simulink model "SVM_test2"  (R2020a)
settings: Solver=VariableStepAuto  StartTime=0.0  StopTime=Inf  FixedStep=Ts/2  RelTol=1e-3
PostLoadFcn:
  | , if any(exist('dsrtsu_mdlpostloadfcn', 'file') ~= 0), dsrtsu_mdlpostloadfcn('Execute', bdroot); end,
InitFcn:
  | , if any(exist('rtifpga_mdlclblib', 'file') ~= 0), rtifpga_mdlclblib('Init', bdroot); end,
model workspace (MAT data in the model file):
  FPGA_SVM_test2_1_Register_1_1_1_write = Simulink.Signal
  FPGA_SVM_test2_1_Register_1_1_1_write.Description = 'RTIFPGA'
  FPGA_SVM_test2_1_Register_1_1_1_write.DataType = 'double'
  FPGA_SVM_test2_1_Register_1_1_1_write.Dimensions = '1'
  FPGA_SVM_test2_1_Register_1_1_1_write.DimensionsMode = 'auto'
  FPGA_SVM_test2_1_Register_1_1_1_write.Complexity = 'auto'
  FPGA_SVM_test2_1_Register_1_1_1_write.SampleTime = -1
  FPGA_SVM_test2_1_Register_1_1_1_write.SamplingMode = 'auto'
  FPGA_SVM_test2_1_Register_2_1_1_write = Simulink.Signal
  FPGA_SVM_test2_1_Register_2_1_1_write.Description = 'RTIFPGA'
  FPGA_SVM_test2_1_Register_2_1_1_write.DataType = 'double'
  FPGA_SVM_test2_1_Register_2_1_1_write.Dimensions = '1'
  FPGA_SVM_test2_1_Register_2_1_1_write.DimensionsMode = 'auto'
  FPGA_SVM_test2_1_Register_2_1_1_write.Complexity = 'auto'
  FPGA_SVM_test2_1_Register_2_1_1_write.SampleTime = -1
  FPGA_SVM_test2_1_Register_2_1_1_write.SamplingMode = 'auto'
  FPGA_SVM_test2_1_Register_3_1_1_write = Simulink.Signal
  FPGA_SVM_test2_1_Register_3_1_1_write.Description = 'RTIFPGA'
  FPGA_SVM_test2_1_Register_3_1_1_write.DataType = 'double'
  FPGA_SVM_test2_1_Register_3_1_1_write.Dimensions = '1'
  FPGA_SVM_test2_1_Register_3_1_1_write.DimensionsMode = 'auto'
  FPGA_SVM_test2_1_Register_3_1_1_write.Complexity = 'auto'
  FPGA_SVM_test2_1_Register_3_1_1_write.SampleTime = -1
  FPGA_SVM_test2_1_Register_3_1_1_write.SamplingMode = 'auto'
  FPGA_SVM_test2_1_Register_4_1_1_write = Simulink.Signal
  FPGA_SVM_test2_1_Register_4_1_1_write.Description = 'RTIFPGA'
  FPGA_SVM_test2_1_Register_4_1_1_write.DataType = 'double'
  FPGA_SVM_test2_1_Register_4_1_1_write.Dimensions = '1'
  FPGA_SVM_test2_1_Register_4_1_1_write.DimensionsMode = 'auto'
  FPGA_SVM_test2_1_Register_4_1_1_write.Complexity = 'auto'
  FPGA_SVM_test2_1_Register_4_1_1_write.SampleTime = -1
  FPGA_SVM_test2_1_Register_4_1_1_write.SamplingMode = 'auto'
  FPGA_SVM_test2_1_Register_5_1_1_write = Simulink.Signal
  FPGA_SVM_test2_1_Register_5_1_1_write.Description = 'RTIFPGA'
  FPGA_SVM_test2_1_Register_5_1_1_write.DataType = 'double'
  FPGA_SVM_test2_1_Register_5_1_1_write.Dimensions = '1'
  FPGA_SVM_test2_1_Register_5_1_1_write.DimensionsMode = 'auto'
  FPGA_SVM_test2_1_Register_5_1_1_write.Complexity = 'auto'
  FPGA_SVM_test2_1_Register_5_1_1_write.SampleTime = -1
  FPGA_SVM_test2_1_Register_5_1_1_write.SamplingMode = 'auto'
  FPGA_SVM_test2_1_Register_6_1_1_write = Simulink.Signal
  FPGA_SVM_test2_1_Register_6_1_1_write.Description = 'RTIFPGA'
  FPGA_SVM_test2_1_Register_6_1_1_write.DataType = 'double'
  FPGA_SVM_test2_1_Register_6_1_1_write.Dimensions = '1'
  FPGA_SVM_test2_1_Register_6_1_1_write.DimensionsMode = 'auto'
  FPGA_SVM_test2_1_Register_6_1_1_write.Complexity = 'auto'
  FPGA_SVM_test2_1_Register_6_1_1_write.SampleTime = -1
  FPGA_SVM_test2_1_Register_6_1_1_write.SamplingMode = 'auto'
  FPGA_SVM_test2_1_Register_7_1_1_write = Simulink.Signal
  FPGA_SVM_test2_1_Register_7_1_1_write.Description = 'RTIFPGA'
  FPGA_SVM_test2_1_Register_7_1_1_write.DataType = 'double'
  FPGA_SVM_test2_1_Register_7_1_1_write.Dimensions = '1'
  FPGA_SVM_test2_1_Register_7_1_1_write.DimensionsMode = 'auto'
  FPGA_SVM_test2_1_Register_7_1_1_write.Complexity = 'auto'
  FPGA_SVM_test2_1_Register_7_1_1_write.SampleTime = -1
  FPGA_SVM_test2_1_Register_7_1_1_write.SamplingMode = 'auto'
values from neighbouring files (symbols this model uses):
  clamp_threshold = 400    [param.m]
  i_fixed_gain = 10*1000/(3*100)    (= 33.3333333333)    [param.m]
  ioa_gain = 1    [param.m]
  ioa_offset = 0.09    [param.m]
  iob_gain = 1    [param.m]
  iob_offset = 0.06    [param.m]
  isa_gain = 1    [param.m]
  isa_offset = 0.1    [param.m]
  isb_gain = 1    [param.m]
  isb_offset = 0.3    [param.m]
  N = 1000    [param.m]
  vca_gain = 1    [param.m]
  vca_offset = 0.8    [param.m]
  vcb_gain = 1    [param.m]
  vcb_offset = 1.7    [param.m]
  vcc_gain = 1    [param.m]
  vcc_offset = 3    [param.m]
  vclamp_gain = 10*(76000+47000)/(3*100*2.5)    (= 1640)    [param.m]
  vclamp_offset = 11.7    [param.m]
  vi_fixed_gain = 10*33000/(3*100*2.5)    (= 440)    [param.m]
  via_gain = 1    [param.m]
  via_offset = 1    [param.m]
  vib_gain = 1    [param.m]
  vib_offset = 0.8    [param.m]
  vic_gain = 1    [param.m]
  vic_offset = -0.35    [param.m]
  voa_fixed_gain = 10*30000/(3*100*2.5)    (= 400)    [param.m]
  voa_gain = 1    [param.m]
  voa_offset = 0.7    [param.m]
libraries: xbsIndex_r4 x466, rti1202lib_adc_class1 x12, rtiproclib x10, simulink x3, rtifpgainterfacelib x1, powerlib_meascontrol x1
(part 1 of 9)
Description:
  | Standard RTI1202 template.
  | Supported MATLAB version:  R2020a.
settings Model: Tag=RTI1202  DSRTSU_INTERNAL_RTI_VER=570  DSRTSU_INTERNAL_RTI_TYPE=rti1202  RTICANMMDATA=struct('GeneralSetupData',struct('modelroot','D:\MarcosGomez\SVM','generalsettings',struct('filesettings',struct('destfolder',struct('Name','RTICANMM_FILES','Check',1),'buildfolder',struct('Name','.','Check',1),'AbsDestfolder',struct('Name','D:\MarcosGomez\SVM\RTICANMM_FILES'),'AbsBuildfolder',struct('Name','D:\MarcosGomez\SVM'))),'options',struct('addpaths',1,'rmpaths',1,'addtrcexclusion',true,'cannavigator',struct('checkmonitoring',0),'show_usrtrc',0,'use_usrtrc',0),'advanced',struct('options',ones(1,100)),'MPSetup',{{}},'RTI',struct('Type','RTI1202','Ver','7.15','Date','02-Nov-2020'),'modelname','SVM_test2','block','SVM_test2'))  DSRTSU_INTERNAL_RTIFPGA=170  OrderedModelArguments=off  Creator=dSPACE2023A  LastModifiedBy=dspace
settings DataIOCC: ReturnWorkspaceOutputs=off
settings OptimizationCC: BlockReduction=off  OptimizeBlockIOStorage=off  BufferReuse=off  GlobalBufferReuse=off  ExpressionFolding=off  LocalBlockOutputs=off  OptimizeDataStoreBuffers=off  BusAssignmentInplaceUpdate=off
settings DebuggingCC: PregeneratedLibrarySubsystemCodeDiagnostic=none  ArithmeticOperatorsInVariantConditions=warning
settings HardwareCC: ProdBitPerPointer=32  ProdBitPerSizeT=32  ProdBitPerPtrDiffT=32  ProdLargestAtomicInteger=Integer  ProdEndianess=BigEndian  ProdWordSize=32  ProdLongLongMode=on  ProdHWDeviceType=Custom Processor->Custom  TargetIntDivRoundTo=Zero  TargetEndianess=BigEndian  TargetHWDeviceType=Custom Processor->Custom
settings ModelReferenceCC: EnableParallelModelReferenceBuilds=on  ParallelModelReferenceMATLABWorkerInit=Load Top Model
settings SFSimCC: SimUseLocalCustomCode=off  MATLABDynamicMemAlloc=off  CustomCodeUndefinedFunction=UseInterfaceOnly
settings RTWCC: Description=dSPACE DS1202 Hardware Platform  SystemTargetFile=rti1202.tlc  MakeCommand=make_rti  TemplateMakefile=rti1202.tmf  RTWUseLocalCustomCode=off
settings CodeAppCC: StateflowObjectComments=on
settings STFCustomTargetCC: ParMdlRefBuildCompliant=on  SystemTargetFile=rti1202.tlc
settings GRTTargetCC: TargetLangStandard=C89/C90 (ANSI)  CompOptLevelCompliant=off  ConcurrentExecutionCompliant=off  CombineOutputUpdateFcns=off  MatFileLogging=off  CPPClassGenCompliant=off  UseToolchainInfoCompliant=off
settings ConfigComp: CovMetricSettings=dswe

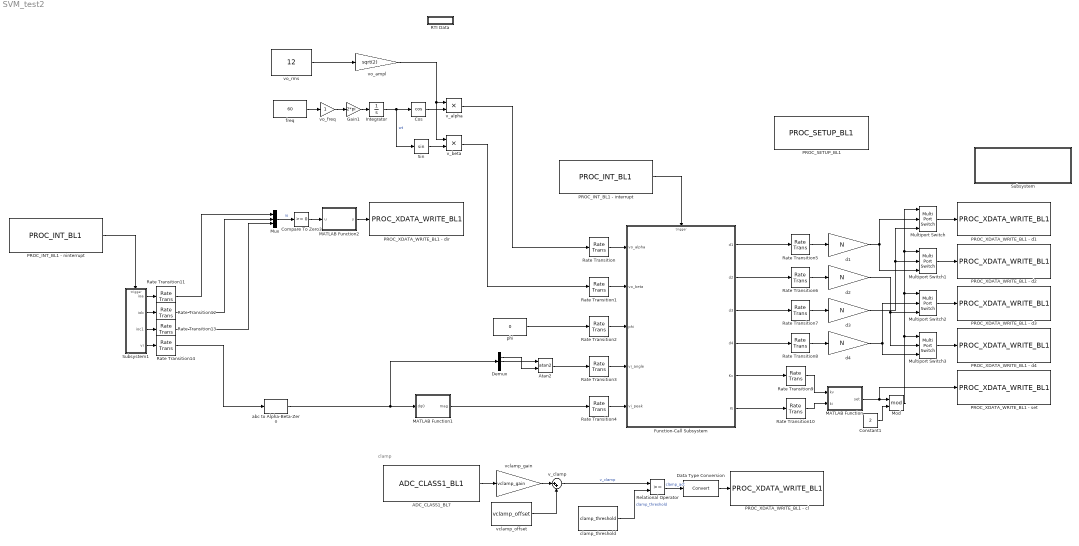
== system SVM_test2 ==
  note: clamp
  ADC_CLASS1_BL7 : rti1202lib_adc_class1/ADC_CLASS1_BL1  DSProperties=struct('RTI',struct('Version',uint32(1),'BlockType',struct('isSLSource',uint8(1),'isSLSink',uint8(1),'isHWSource',uint8(0),'isHWSink',uint8(1),'isSetup',uint8(0),'isInline',uint8(1),'isNonInline',uint8(0),'isInterrupt',uint8(0),'isChannelwise',uint8(1)),'IOBoardType',{{'DS120X','STD','ADCC1'}},'UnitType','ADC','Identifier','ADC','DialogType','ML','BlockSet','NONE','SlaveProcessor','NONE'))  RTIBlockInterface=struct('InputPortsActive',0,'InputPortsWidth',int32(1),'InputPortsDataType',{{'SS_BOOLEAN'}},'InputPortsName',{{'Continue'}},'OutputPortsActive',[1 0],'OutputPortsWidth',int32([1 1]),'OutputPortsDataType',{{'SS_DOUBLE','SS_INT16'}},'OutputPortsName',{{'ADC','Status'}},'DialogFcn','rti120xstdadcc1adcgui','SampleTime',{{-1}},'InitLevel',3,'IconTransparency','on','BlockDisplay',{{['ADC CL1\nChannel: 7'],'center'}},'BlockName',struct('Token',{{'ADC_CLASS1_BL1'}}))  RTIBlockParameters=struct('ReadMode',{{1,'OFF',[1 2]}},'ChannelNo',{{7,'OFF',[]}},'ConversionMode',{{1,'OFF',[1 2]}},'TriggerSource',{{1,'OFF',[1 2]}},'TriggerLineIn',{{1,'OFF',[1 16]}},'SampleMode',{{1,'OFF',[1 2]}},'BurstTriggerSource',{{1,'OFF',[1 2]}},'BurstTriggerLine',{{1,'OFF',[1 16]}},'ConvTriggerSource',{{3,'OFF',[1 3]}},'ConvTriggerLine',{{1,'OFF',[1 16]}},'ConvPeriod',{{'100e-6','OFF',[1e-6 1.34]}},'ConvPeriodCheck',{{0,'OFF',[]}},'BurstSize',{{'10','OFF',[]}},'BurstSizeCheck',{{0,'OFF',[]}},'DataSetOffset',{{'0','OFF',[]}},'DataSetOffsetCheck',{{0,'OFF',[]}},'DataSetLength',{{'1','OFF',[]}},'DataSetLengthCheck',{{0,'OFF',[]}},'EnableTriggerEvent',{{0,'OFF',[0 1]}},'TriggerMode',{{2,'OFF',[1 3]}},'TriggerLineOut',{{1,'OFF',[1 16]}},'ADCSWStartEnable',{{0,'OFF',[0 1]}},'SampleTime',{{'-1','OFF',[-1 inf]}},'SampleTimeCheck',{{1,'OFF',[]}},'StatusPortEnable',{{0,'OFF',[0 1]}},'TLCFileName',{{'rti120xadc_c1_adc','OFF',[]}})  RTISFcnParameters=struct('ReadMode','int16','ChannelNo','int16','ConversionMode','int16','TriggerSource','int16','TriggerLineIn','int16','SampleMode','int16','BurstTriggerSource','int16','BurstTriggerLine','int16','ConvTriggerSource','int16','ConvTriggerLine','int16','ConvPeriod','double','BurstSize','int16','DataSetOffset','int16','DataSetLength','int16','EnableTriggerEvent','int16','TriggerMode','int16','TriggerLineOut','int16','ADCSWStartEnable','int16','SampleTime','double','StatusPortEnable','int16','TLCFileName','char')  RTIBlockParaDefault=struct('ReadMode',1,'ChannelNo',1,'ConversionMode',1,'TriggerSource',1,'TriggerLineIn',1,'SampleMode',1,'BurstTriggerSource',1,'BurstTriggerLine',1,'ConvTriggerSource',3,'ConvTriggerLine',1,'ConvPeriod',0.0001,'ConvPeriodCheck',0,'BurstSize',10,'BurstSizeCheck',0,'DataSetOffset',0,'DataSetOffsetCheck',0,'DataSetLength',1,'DataSetLengthCheck',0,'EnableTriggerEvent',0,'TriggerMode',2,'TriggerLineOut',1,'ADCSWStartEnable',0,'SampleTime',-1,'SampleTimeCheck',1,'StatusPortEnable',0,'TLCFileName','rti120xadc_c1_adc')
  Atan2 : Trigonometry  Operator=atan2
  Compare To Zero3 : simulink/Logic and Bit Operations/Compare To Zero  relop=>=  OutDataTypeStr=boolean
  Constant1 : Constant  Value=2
  Cos : Trigonometry  Operator=cos
  Data Type Conversion : DataTypeConversion
  Demux : Demux  Outputs=3
  Function-Call Subsystem : Subsystem  TreatAsAtomicUnit=on
  Gain1 : Gain  Gain=2*pi
  Integrator : Integrator
  MATLAB Function : MATLAB Function  TreatAsAtomicUnit=on
  MATLAB Function1 : MATLAB Function  TreatAsAtomicUnit=on
  MATLAB Function2 : MATLAB Function  TreatAsAtomicUnit=on
  Mod : Math  Operator=mod  SaturateOnIntegerOverflow=on
  Multiport Switch{,1..3} (4 alike) : MultiPortSwitch  DataPortOrder=Zero-based contiguous  Inputs=2  zeroidx=on
  Mux : Mux  Inputs=3
  PROC_INT_BL1 - interrupt : rtiproclib/PROC_INT_BL1  DSProperties=struct('RTI',struct('Version',uint32(4),'BlockType',struct('isSLSource',uint8(1),'isSLSink',uint8(0),'isHWSource',uint8(0),'isHWSink',uint8(0),'isSetup',uint8(1),'isInline',uint8(1),'isNonInline',uint8(0),'isInterrupt',uint8(0),'isChannelwise',uint8(0)),'IOBoardType','DSPROC','UnitType','','Identifier','INT','DialogType','ML','BlockSet','DSPROC','SlaveProcessor',''))  RTIBlockInterface=struct('OutputPortsActive',1,'OutputPortsWidth',int32(1),'OutputPortsName',{{'Interrupt'}},'FunctionCall',uint32(0),'DialogFcn','rtiprocintgui','InitLevel',3,'BlockDisplay',{{['Interrupt In 1\ninterrupt \nBoard: 1'],'center'}},'IconTransparency','on','BlockName',struct('Token',{{'PROC_INT_BL1'}}))  RTIBlockParameters=struct('BoardNo',{{'1','OFF',[1 16]}},'ChannelNo',{{'1','OFF',[1 8]}},'AccessTyp',{{'Interrupt','OFF',[]}},'BinaryPoint',{{'0','OFF',[]}},'DataFormat',{{'unsigned','OFF',[]}},'BufferLength',{{'0','OFF',[]}},'MultiChAccess',{{'0','OFF',[]}},'ModelPortBlock',{{{struct('BlockId','','SignalId','')},'OFF',[]}})  RTISFcnParameters=struct('BoardNo','double','ChannelNo','double','AccessTyp','char','BinaryPoint','double','DataFormat','char','BufferLength','double')  RTIBlockParaDefault=struct('BoardNo','1','ChannelNo','1','AccessTyp','Interrupt','BinaryPoint','10','DataFormat','unsigned','BufferLength','0','MultiChAccess','0','ModelPortBlock',{{struct('BlockId','','SignalId','')}})
  PROC_INT_BL1 - ninterrupt : rtiproclib/PROC_INT_BL1  DSProperties=struct('RTI',struct('Version',uint32(4),'BlockType',struct('isSLSource',uint8(1),'isSLSink',uint8(0),'isHWSource',uint8(0),'isHWSink',uint8(0),'isSetup',uint8(1),'isInline',uint8(1),'isNonInline',uint8(0),'isInterrupt',uint8(0),'isChannelwise',uint8(0)),'IOBoardType','DSPROC','UnitType','','Identifier','INT','DialogType','ML','BlockSet','DSPROC','SlaveProcessor',''))  RTIBlockInterface=struct('OutputPortsActive',1,'OutputPortsWidth',int32(1),'OutputPortsName',{{'Interrupt'}},'FunctionCall',uint32(0),'DialogFcn','rtiprocintgui','InitLevel',3,'BlockDisplay',{{['Interrupt In 2\nninterrupt \nBoard: 1'],'center'}},'IconTransparency','on','BlockName',struct('Token',{{'PROC_INT_BL1'}}))  RTIBlockParameters=struct('BoardNo',{{'1','OFF',[1 16]}},'ChannelNo',{{'2','OFF',[1 8]}},'AccessTyp',{{'Interrupt','OFF',[]}},'BinaryPoint',{{'0','OFF',[]}},'DataFormat',{{'unsigned','OFF',[]}},'BufferLength',{{'0','OFF',[]}},'MultiChAccess',{{'0','OFF',[]}},'ModelPortBlock',{{{struct('BlockId','','SignalId','')},'OFF',[]}})  RTISFcnParameters=struct('BoardNo','double','ChannelNo','double','AccessTyp','char','BinaryPoint','double','DataFormat','char','BufferLength','double')  RTIBlockParaDefault=struct('BoardNo','1','ChannelNo','1','AccessTyp','Interrupt','BinaryPoint','10','DataFormat','unsigned','BufferLength','0','MultiChAccess','0','ModelPortBlock',{{struct('BlockId','','SignalId','')}})
  PROC_SETUP_BL1 : rtiproclib/PROC_SETUP_BL1  DSProperties=struct('RTI',struct('Version',uint32(3),'BlockType',struct('isSLSource',uint8(0),'isSLSink',uint8(0),'isHWSource',uint8(0),'isHWSink',uint8(0),'isSetup',uint8(1),'isInline',uint8(1),'isNonInline',uint8(0),'isInterrupt',uint8(0),'isChannelwise',uint8(0)),'IOBoardType','DSPROC','UnitType','SETUP','Identifier','SETUP','DialogType','ML','BlockSet','NONE','SlaveProcessor',''))  RTIBlockInterface=struct('OutputPortsWidth',int32(0),'OutputPortsActive',0,'InitLevel',3,'DialogFcn','rtiprocsetupgui','BlockDisplay',{{['Processor Setup'],'auto'}},'IconTransparency','off','BlockName',struct('Token',{{'PROC_SETUP_BL1'}}))  RTIBlockParameters=struct('NumBoardsUsed',{{1,'OFF',[1 16]}},'ModelMode',{{1,'OFF',[]}},'IniFileList',{{struct('Fullname','','Filename','','Relname','','Assigned',0),'OFF',[]}},'SubsysList',{{struct('SharedAccess',1,'SetupBlockHandle',23837.00439453125,'SetupBlockName','FPGA_SETUP_BL1','SubsysName','Subsystem','SubsysHandle',14037.020629882813,'SubsysPath','/Subsystem','Assigned',1,'IniFilePath','D:\MarcosGomez\SVM\SVM_test2_rtiFPGA/INI/Subsystem_96F06F45D83184.ini','IniFileName','Subsystem_96F06F45D83184','IniFileDate',739590.85696759261),'OFF',[]}},'AssignList',{{struct('BoardNumber',{1,2,3,4,5,6,7,8,9,10,11,12,13,14,15,16},'ModelType',{1,0,0,0,0,0,0,0,0,0,0,0,0,0,0,0},'ModelNo',{1,0,0,0,0,0,0,0,0,0,0,0,0,0,0,0},'ProgOption',{2,0,0,0,0,0,0,0,0,0,0,0,0,0,0,0},'IncludeBuild',{1,0,0,0,0,0,0,0,0,0,0,0,0,0,0,0},'IncludeProcAppl',{true,0,0,0,0,0,0,0,0,0,0,0,0,0,0,0}),'OFF',[]}},'ProcSetupHandles',{{-1,'OFF',[]}},'MaxNumBoards',{{16,'OFF',[]}},'ModelPath',{{'D:\MarcosGomez\SVM','OFF',[]}},'FrameDir',{{[' '],'OFF',[]}},'TLCFileName',{{'rtiprocsetup','OFF',[]}},'IsNewBlock',{{0,'OFF',[]}},'NeedsCodeGen',{{0,'OFF',[]}})  RTISFcnParameters=struct('FrameDir','char','TLCFileName','char')  RTIBlockParaDefault=struct('NumBoardsUsed',1,'ModelMode',1,'IniFileList',struct('Fullname','','Filename','','Relname','','Assigned',''),'SubsysList',struct('SubsysName','','SubsysPath','','SubsysHandle','','SetupBlockHandle','','SetupBlockName','','Filename','','Relname','','IniFilePath','','IniFileName','','IniFileDate','','Assigned',''),'AssignList',struct('BoardNumber','','ModelType','','ModelNo','','ProgOption','','IncludeBuild','','IncludeProcAppl',''),'ProcSetupHandles',-1,'MaxNumBoards',16,'ModelPath',[' '],'FrameDir',[' '],'TLCFileName','rtiprocsetup','IsNewBlock',1,'NeedsCodeGen',0)
      settings: AttributesFormatString=FPGA-Build / Offline Simulation
  PROC_XDATA_WRITE_BL1 - cl : rtiproclib/PROC_XDATA_WRITE_BL1  DSProperties=struct('RTI',struct('Version',uint32(6),'BlockType',struct('isSLSource',uint8(0),'isSLSink',uint8(1),'isHWSource',uint8(0),'isHWSink',uint8(0),'isSetup',uint8(0),'isInline',uint8(1),'isNonInline',uint8(0),'isInterrupt',uint8(0),'isChannelwise',uint8(0)),'IOBoardType','DSPROC','UnitType','','Identifier','PHSWRITE','DialogType','ML','BlockSet','DSPROC','SlaveProcessor',''))  RTIBlockInterface=struct('InputPortsActive',true,'InputPortsWidth',{{'DYNAMICALLY_SIZED'}},'InputPortsDataType',{{'SS_DOUBLE'}},'InputPortsName',{{'Data'}},'InitLevel',3,'DialogFcn','rtiprocphswritegui','BlockDisplay',{{['Register Out 3\ncl\nGroup: 1 Board: 1'],'auto'}},'IconTransparency','on','BlockName',struct('Token',{{'PROC_XDATA_WRITE_BL1'}}))  RTIBlockParameters=struct('BoardNo',{{'1','OFF',[1 16]}},'ChannelNo',{{'3','OFF',[]}},'AccessTyp',{{'Register','OFF',[]}},'BinaryPoint',{{'0','OFF',[]}},'DataFormat',{{'unsigned','OFF',[]}},'BufferLength',{{'0','OFF',[]}},'GroupNo',{{'1','OFF',[]}},'MultiChAccess',{{'0','OFF',[]}},'InitOnly',{{'0','OFF',[]}},'InitValue',{{'0','OFF',[]}},'TLCFileName',{{'rtiprocphswrite','OFF',[]}},'ModelPortBlock',{{{struct('BlockId','','SignalId','')},'OFF',[]}})  RTISFcnParameters=struct('BoardNo','double','ChannelNo','double','GroupNo','double','AccessTyp','char','BinaryPoint','double','DataFormat','char','BufferLength','double','InitOnly','double','InitValue','double','TLCFileName','char')  RTIBlockParaDefault=struct('BoardNo','1','ChannelNo','0','AccessTyp','Register','BinaryPoint','10','DataFormat','signed','BufferLength','16','GroupNo','0','MultiChAccess','0','InitOnly','0','InitValue','0','TLCFileName','rtiprocphswrite','ModelPortBlock',{{struct('BlockId','','SignalId','','BusObject','')}})
  PROC_XDATA_WRITE_BL1 - d1 : rtiproclib/PROC_XDATA_WRITE_BL1  DSProperties=struct('RTI',struct('Version',uint32(6),'BlockType',struct('isSLSource',uint8(0),'isSLSink',uint8(1),'isHWSource',uint8(0),'isHWSink',uint8(0),'isSetup',uint8(0),'isInline',uint8(1),'isNonInline',uint8(0),'isInterrupt',uint8(0),'isChannelwise',uint8(0)),'IOBoardType','DSPROC','UnitType','','Identifier','PHSWRITE','DialogType','ML','BlockSet','DSPROC','SlaveProcessor',''))  RTIBlockInterface=struct('InputPortsActive',true,'InputPortsWidth',{{'DYNAMICALLY_SIZED'}},'InputPortsDataType',{{'SS_DOUBLE'}},'InputPortsName',{{'Data'}},'InitLevel',3,'DialogFcn','rtiprocphswritegui','BlockDisplay',{{['Register Out 4\nd1\nGroup: 1 Board: 1'],'auto'}},'IconTransparency','on','BlockName',struct('Token',{{'PROC_XDATA_WRITE_BL1'}}))  RTIBlockParameters=struct('BoardNo',{{'1','OFF',[1 16]}},'ChannelNo',{{'4','OFF',[]}},'AccessTyp',{{'Register','OFF',[]}},'BinaryPoint',{{'0','OFF',[]}},'DataFormat',{{'unsigned','OFF',[]}},'BufferLength',{{'0','OFF',[]}},'GroupNo',{{'1','OFF',[]}},'MultiChAccess',{{'0','OFF',[]}},'InitOnly',{{'0','OFF',[]}},'InitValue',{{'0','OFF',[]}},'TLCFileName',{{'rtiprocphswrite','OFF',[]}},'ModelPortBlock',{{{struct('BlockId','','SignalId','')},'OFF',[]}})  RTISFcnParameters=struct('BoardNo','double','ChannelNo','double','GroupNo','double','AccessTyp','char','BinaryPoint','double','DataFormat','char','BufferLength','double','InitOnly','double','InitValue','double','TLCFileName','char')  RTIBlockParaDefault=struct('BoardNo','1','ChannelNo','0','AccessTyp','Register','BinaryPoint','10','DataFormat','signed','BufferLength','16','GroupNo','0','MultiChAccess','0','InitOnly','0','InitValue','0','TLCFileName','rtiprocphswrite','ModelPortBlock',{{struct('BlockId','','SignalId','','BusObject','')}})
  PROC_XDATA_WRITE_BL1 - d2 : rtiproclib/PROC_XDATA_WRITE_BL1  DSProperties=struct('RTI',struct('Version',uint32(6),'BlockType',struct('isSLSource',uint8(0),'isSLSink',uint8(1),'isHWSource',uint8(0),'isHWSink',uint8(0),'isSetup',uint8(0),'isInline',uint8(1),'isNonInline',uint8(0),'isInterrupt',uint8(0),'isChannelwise',uint8(0)),'IOBoardType','DSPROC','UnitType','','Identifier','PHSWRITE','DialogType','ML','BlockSet','DSPROC','SlaveProcessor',''))  RTIBlockInterface=struct('InputPortsActive',true,'InputPortsWidth',{{'DYNAMICALLY_SIZED'}},'InputPortsDataType',{{'SS_DOUBLE'}},'InputPortsName',{{'Data'}},'InitLevel',3,'DialogFcn','rtiprocphswritegui','BlockDisplay',{{['Register Out 5\nd2\nGroup: 1 Board: 1'],'auto'}},'IconTransparency','on','BlockName',struct('Token',{{'PROC_XDATA_WRITE_BL1'}}))  RTIBlockParameters=struct('BoardNo',{{'1','OFF',[1 16]}},'ChannelNo',{{'5','OFF',[]}},'AccessTyp',{{'Register','OFF',[]}},'BinaryPoint',{{'0','OFF',[]}},'DataFormat',{{'unsigned','OFF',[]}},'BufferLength',{{'0','OFF',[]}},'GroupNo',{{'1','OFF',[]}},'MultiChAccess',{{'0','OFF',[]}},'InitOnly',{{'0','OFF',[]}},'InitValue',{{'0','OFF',[]}},'TLCFileName',{{'rtiprocphswrite','OFF',[]}},'ModelPortBlock',{{{struct('BlockId','','SignalId','')},'OFF',[]}})  RTISFcnParameters=struct('BoardNo','double','ChannelNo','double','GroupNo','double','AccessTyp','char','BinaryPoint','double','DataFormat','char','BufferLength','double','InitOnly','double','InitValue','double','TLCFileName','char')  RTIBlockParaDefault=struct('BoardNo','1','ChannelNo','0','AccessTyp','Register','BinaryPoint','10','DataFormat','signed','BufferLength','16','GroupNo','0','MultiChAccess','0','InitOnly','0','InitValue','0','TLCFileName','rtiprocphswrite','ModelPortBlock',{{struct('BlockId','','SignalId','','BusObject','')}})
  PROC_XDATA_WRITE_BL1 - d3 : rtiproclib/PROC_XDATA_WRITE_BL1  DSProperties=struct('RTI',struct('Version',uint32(6),'BlockType',struct('isSLSource',uint8(0),'isSLSink',uint8(1),'isHWSource',uint8(0),'isHWSink',uint8(0),'isSetup',uint8(0),'isInline',uint8(1),'isNonInline',uint8(0),'isInterrupt',uint8(0),'isChannelwise',uint8(0)),'IOBoardType','DSPROC','UnitType','','Identifier','PHSWRITE','DialogType','ML','BlockSet','DSPROC','SlaveProcessor',''))  RTIBlockInterface=struct('InputPortsActive',true,'InputPortsWidth',{{'DYNAMICALLY_SIZED'}},'InputPortsDataType',{{'SS_DOUBLE'}},'InputPortsName',{{'Data'}},'InitLevel',3,'DialogFcn','rtiprocphswritegui','BlockDisplay',{{['Register Out 6\nd3\nGroup: 1 Board: 1'],'auto'}},'IconTransparency','on','BlockName',struct('Token',{{'PROC_XDATA_WRITE_BL1'}}))  RTIBlockParameters=struct('BoardNo',{{'1','OFF',[1 16]}},'ChannelNo',{{'6','OFF',[]}},'AccessTyp',{{'Register','OFF',[]}},'BinaryPoint',{{'0','OFF',[]}},'DataFormat',{{'unsigned','OFF',[]}},'BufferLength',{{'0','OFF',[]}},'GroupNo',{{'1','OFF',[]}},'MultiChAccess',{{'0','OFF',[]}},'InitOnly',{{'0','OFF',[]}},'InitValue',{{'0','OFF',[]}},'TLCFileName',{{'rtiprocphswrite','OFF',[]}},'ModelPortBlock',{{{struct('BlockId','','SignalId','')},'OFF',[]}})  RTISFcnParameters=struct('BoardNo','double','ChannelNo','double','GroupNo','double','AccessTyp','char','BinaryPoint','double','DataFormat','char','BufferLength','double','InitOnly','double','InitValue','double','TLCFileName','char')  RTIBlockParaDefault=struct('BoardNo','1','ChannelNo','0','AccessTyp','Register','BinaryPoint','10','DataFormat','signed','BufferLength','16','GroupNo','0','MultiChAccess','0','InitOnly','0','InitValue','0','TLCFileName','rtiprocphswrite','ModelPortBlock',{{struct('BlockId','','SignalId','','BusObject','')}})
  PROC_XDATA_WRITE_BL1 - d4 : rtiproclib/PROC_XDATA_WRITE_BL1  DSProperties=struct('RTI',struct('Version',uint32(6),'BlockType',struct('isSLSource',uint8(0),'isSLSink',uint8(1),'isHWSource',uint8(0),'isHWSink',uint8(0),'isSetup',uint8(0),'isInline',uint8(1),'isNonInline',uint8(0),'isInterrupt',uint8(0),'isChannelwise',uint8(0)),'IOBoardType','DSPROC','UnitType','','Identifier','PHSWRITE','DialogType','ML','BlockSet','DSPROC','SlaveProcessor',''))  RTIBlockInterface=struct('InputPortsActive',true,'InputPortsWidth',{{'DYNAMICALLY_SIZED'}},'InputPortsDataType',{{'SS_DOUBLE'}},'InputPortsName',{{'Data'}},'InitLevel',3,'DialogFcn','rtiprocphswritegui','BlockDisplay',{{['Register Out 7\nd4\nGroup: 1 Board: 1'],'auto'}},'IconTransparency','on','BlockName',struct('Token',{{'PROC_XDATA_WRITE_BL1'}}))  RTIBlockParameters=struct('BoardNo',{{'1','OFF',[1 16]}},'ChannelNo',{{'7','OFF',[]}},'AccessTyp',{{'Register','OFF',[]}},'BinaryPoint',{{'0','OFF',[]}},'DataFormat',{{'unsigned','OFF',[]}},'BufferLength',{{'0','OFF',[]}},'GroupNo',{{'1','OFF',[]}},'MultiChAccess',{{'0','OFF',[]}},'InitOnly',{{'0','OFF',[]}},'InitValue',{{'0','OFF',[]}},'TLCFileName',{{'rtiprocphswrite','OFF',[]}},'ModelPortBlock',{{{struct('BlockId','','SignalId','')},'OFF',[]}})  RTISFcnParameters=struct('BoardNo','double','ChannelNo','double','GroupNo','double','AccessTyp','char','BinaryPoint','double','DataFormat','char','BufferLength','double','InitOnly','double','InitValue','double','TLCFileName','char')  RTIBlockParaDefault=struct('BoardNo','1','ChannelNo','0','AccessTyp','Register','BinaryPoint','10','DataFormat','signed','BufferLength','16','GroupNo','0','MultiChAccess','0','InitOnly','0','InitValue','0','TLCFileName','rtiprocphswrite','ModelPortBlock',{{struct('BlockId','','SignalId','','BusObject','')}})
  PROC_XDATA_WRITE_BL1 - dir : rtiproclib/PROC_XDATA_WRITE_BL1  DSProperties=struct('RTI',struct('Version',uint32(6),'BlockType',struct('isSLSource',uint8(0),'isSLSink',uint8(1),'isHWSource',uint8(0),'isHWSink',uint8(0),'isSetup',uint8(0),'isInline',uint8(1),'isNonInline',uint8(0),'isInterrupt',uint8(0),'isChannelwise',uint8(0)),'IOBoardType','DSPROC','UnitType','','Identifier','PHSWRITE','DialogType','ML','BlockSet','DSPROC','SlaveProcessor',''))  RTIBlockInterface=struct('InputPortsActive',true,'InputPortsWidth',{{'DYNAMICALLY_SIZED'}},'InputPortsDataType',{{'SS_DOUBLE'}},'InputPortsName',{{'Data'}},'InitLevel',3,'DialogFcn','rtiprocphswritegui','BlockDisplay',{{['Register Out 2\ndir \nGroup: 1 Board: 1'],'auto'}},'IconTransparency','on','BlockName',struct('Token',{{'PROC_XDATA_WRITE_BL1'}}))  RTIBlockParameters=struct('BoardNo',{{'1','OFF',[1 16]}},'ChannelNo',{{'2','OFF',[]}},'AccessTyp',{{'Register','OFF',[]}},'BinaryPoint',{{'0','OFF',[]}},'DataFormat',{{'unsigned','OFF',[]}},'BufferLength',{{'0','OFF',[]}},'GroupNo',{{'1','OFF',[]}},'MultiChAccess',{{'0','OFF',[]}},'InitOnly',{{'0','OFF',[]}},'InitValue',{{'0','OFF',[]}},'TLCFileName',{{'rtiprocphswrite','OFF',[]}},'ModelPortBlock',{{{struct('BlockId','','SignalId','')},'OFF',[]}})  RTISFcnParameters=struct('BoardNo','double','ChannelNo','double','GroupNo','double','AccessTyp','char','BinaryPoint','double','DataFormat','char','BufferLength','double','InitOnly','double','InitValue','double','TLCFileName','char')  RTIBlockParaDefault=struct('BoardNo','1','ChannelNo','0','AccessTyp','Register','BinaryPoint','10','DataFormat','signed','BufferLength','16','GroupNo','0','MultiChAccess','0','InitOnly','0','InitValue','0','TLCFileName','rtiprocphswrite','ModelPortBlock',{{struct('BlockId','','SignalId','','BusObject','')}})
  PROC_XDATA_WRITE_BL1 - set : rtiproclib/PROC_XDATA_WRITE_BL1  DSProperties=struct('RTI',struct('Version',uint32(6),'BlockType',struct('isSLSource',uint8(0),'isSLSink',uint8(1),'isHWSource',uint8(0),'isHWSink',uint8(0),'isSetup',uint8(0),'isInline',uint8(1),'isNonInline',uint8(0),'isInterrupt',uint8(0),'isChannelwise',uint8(0)),'IOBoardType','DSPROC','UnitType','','Identifier','PHSWRITE','DialogType','ML','BlockSet','DSPROC','SlaveProcessor',''))  RTIBlockInterface=struct('InputPortsActive',true,'InputPortsWidth',{{'DYNAMICALLY_SIZED'}},'InputPortsDataType',{{'SS_DOUBLE'}},'InputPortsName',{{'Data'}},'InitLevel',3,'DialogFcn','rtiprocphswritegui','BlockDisplay',{{['Register Out 1\nset\nGroup: 1 Board: 1'],'auto'}},'IconTransparency','on','BlockName',struct('Token',{{'PROC_XDATA_WRITE_BL1'}}))  RTIBlockParameters=struct('BoardNo',{{'1','OFF',[1 16]}},'ChannelNo',{{'1','OFF',[]}},'AccessTyp',{{'Register','OFF',[]}},'BinaryPoint',{{'0','OFF',[]}},'DataFormat',{{'unsigned','OFF',[]}},'BufferLength',{{'0','OFF',[]}},'GroupNo',{{'1','OFF',[]}},'MultiChAccess',{{'0','OFF',[]}},'InitOnly',{{'0','OFF',[]}},'InitValue',{{'0','OFF',[]}},'TLCFileName',{{'rtiprocphswrite','OFF',[]}},'ModelPortBlock',{{{struct('BlockId','','SignalId','')},'OFF',[]}})  RTISFcnParameters=struct('BoardNo','double','ChannelNo','double','GroupNo','double','AccessTyp','char','BinaryPoint','double','DataFormat','char','BufferLength','double','InitOnly','double','InitValue','double','TLCFileName','char')  RTIBlockParaDefault=struct('BoardNo','1','ChannelNo','0','AccessTyp','Register','BinaryPoint','10','DataFormat','signed','BufferLength','16','GroupNo','0','MultiChAccess','0','InitOnly','0','InitValue','0','TLCFileName','rtiprocphswrite','ModelPortBlock',{{struct('BlockId','','SignalId','','BusObject','')}})
  RTI Data : Subsystem  Tag=struct('RTIDataServer',struct('RTIDataServerVs','2','RTIModelDescription','struct(''main'',''SVM_test2'',''sub'','''',''isMp'',0)'))  LoadFcn="if exist('rtidc'), try,  rtidc('DataHostBlockClbLoad', gcbh); catch, disp(['Warning: ''LoadFcn'' for RTI Data block failed: ' lasterr]); end, end,"  mask(RTI_DATA_HOST){}
      mask help:
      | RTI Data Block.
      | This block is used by RTI to store internal model-dependent data.
      | Please keep this block on the root level of the model. Deleting this block will result in data loss.
      |
      | NEVER DELETE OR COPY THIS BLOCK!
      settings: CopyFcn="if exist('rtidc'), try,  rtidc('DataHostBlockClbCopy', gcbh); catch, disp(['Warning: ''CopyFcn'' for RTI Data block failed: ' lasterr]); end, end,"  DeleteFcn="if exist('rtidc'), try,  rtidc('DataHostBlockClbDelete', gcbh); catch, disp(['Warning: ''DeleteFcn'' for RTI Data block failed: ' lasterr]); end, end,"  ModelCloseFcn="if exist('rtidc'), try,  rtidc('DataHostBlockClbModelClose', gcbh); catch, disp(['Warning: ''ModelCloseFcn'' for RTI Data block failed: ' lasterr]); end, end,"  PreSaveFcn="if exist('rtidc'), try,  rtidc('DataHostBlockClbPreSave', gcbh); catch, disp(['Warning: ''PreSaveFcn'' for RTI Data block failed: ' lasterr]); end, end,"  PostSaveFcn="if exist('rtidc'), try,  rtidc('DataHostBlockClbPostSave', gcbh); catch, disp(['Warning: ''PostSaveFcn'' for RTI Data block failed: ' lasterr]); end, end,"  NameChangeFcn="if exist('rtidc'), try,  rtidc('DataHostBlockClbNameChange', gcbh); catch, disp(['Warning: ''NameChangeFcn'' for RTI Data block failed: ' lasterr]); end, end,"
      mask Help:
      | RTI Data Block.
      | This block is used by RTI to store internal model-dependent data.
      | Please keep this block on the root level of the model. Deleting this block will result in data loss.
      | 
      | NEVER DELETE OR COPY THIS BLOCK!
      mask Display:
      | text(0.5, 0.5, 'RTI Data', 'HorizontalAlignment', 'center');
      | plot([1 0]);
  Rate Transition{,1..14} (15 alike) : RateTransition  Deterministic=off
  Relational Operator : RelationalOperator  OutDataTypeStr=boolean  RndMeth=Simplest
  Sin : Trigonometry
  Subsystem : Subsystem
  Subsystem1 : Subsystem
  abc to Alpha-Beta-Zero : powerlib_meascontrol/Transformations/abc to Alpha-Beta-Zero
  clamp_threshold : Constant  Value=clamp_threshold
  d{1..4} (4 alike) : Gain  Gain=N
  freq : Constant  Value=60
  phi : Constant  Value=0
  v_alpha : Product
  v_beta : Product
  v_clamp : Sum  Inputs=|++
  vclamp_gain : Gain  Gain=vclamp_gain
  vclamp_offset : Constant  Value=vclamp_offset
  vo_ampl : Gain  Gain=sqrt(2)
  vo_freq : Gain
  vo_rms : Constant  Value=12
  wires:
  ADC_CLASS1_BL7/1 -> vclamp_gain/1
  vclamp_offset/1 -> v_clamp/2
  Function-Call Subsystem/4(d4) -> Rate Transition8/1
  Data Type Conversion/1 -> PROC_XDATA_WRITE_BL1 - cl/1
  Function-Call Subsystem/5(Kv) -> Rate Transition9/1
  Function-Call Subsystem/2(d2) -> Rate Transition6/1
  Function-Call Subsystem/1(d1) -> Rate Transition5/1
  Function-Call Subsystem/6(Ki) -> Rate Transition10/1
  Rate Transition7/1 -> d3/1
  Rate Transition6/1 -> d2/1
  Rate Transition5/1 -> d1/1
  Rate Transition10/1 -> MATLAB Function/2(ki)
  Rate Transition1/1 -> Function-Call Subsystem/2(vo_beta)
  Rate Transition8/1 -> d4/1
  Rate Transition4/1 -> Function-Call Subsystem/5(vi_peak)
  Rate Transition/1 -> Function-Call Subsystem/1(vo_alpha)
  Rate Transition9/1 -> MATLAB Function/1(kv)
  Mux/1 -> Compare To Zero3/1  "io"
  clamp_threshold/1 -> Relational Operator/2  "clamp_threshold"
  d1/1 -> Multiport Switch1/3, Multiport Switch/2
  d4/1 -> Multiport Switch2/2, Multiport Switch3/3
  Rate Transition2/1 -> Function-Call Subsystem/3(phi)
  d3/1 -> Multiport Switch/3, Multiport Switch1/2
  d2/1 -> Multiport Switch3/2, Multiport Switch2/3
  PROC_INT_BL1 - interrupt/1 -> Function-Call Subsystem/Trigger
  phi/1 -> Rate Transition2/1
  vo_rms/1 -> vo_ampl/1
  v_alpha/1 -> Rate Transition/1
  Cos/1 -> v_alpha/2
  vclamp_gain/1 -> v_clamp/1
  MATLAB Function2/1(y) -> PROC_XDATA_WRITE_BL1 - dir/1
  Integrator/1 -> Sin/1, Cos/1  "wt"
  Function-Call Subsystem/3(d3) -> Rate Transition7/1
  v_clamp/1 -> Relational Operator/1  "v_clamp"
  Sin/1 -> v_beta/2
  Gain1/1 -> Integrator/1
  Relational Operator/1 -> Data Type Conversion/1  "clamp_act"
  v_beta/1 -> Rate Transition1/1
  Compare To Zero3/1 -> MATLAB Function2/1(u)
  Rate Transition3/1 -> Function-Call Subsystem/4(vi_angle)
  freq/1 -> vo_freq/1
  MATLAB Function/1(set) -> PROC_XDATA_WRITE_BL1 - set/1, Mod/1
  abc to Alpha-Beta-Zero/1 -> MATLAB Function1/1(dq0), Demux/1
  Demux/1 -> Atan2/2
  Demux/2 -> Atan2/1
  Atan2/1 -> Rate Transition3/1
  MATLAB Function1/1(mag) -> Rate Transition4/1
  Multiport Switch/1 -> PROC_XDATA_WRITE_BL1 - d1/1
  Multiport Switch1/1 -> PROC_XDATA_WRITE_BL1 - d2/1
  Multiport Switch2/1 -> PROC_XDATA_WRITE_BL1 - d3/1
  Multiport Switch3/1 -> PROC_XDATA_WRITE_BL1 - d4/1
  Constant1/1 -> Mod/2
  Mod/1 -> Multiport Switch3/1, Multiport Switch/1, Multiport Switch1/1, Multiport Switch2/1
  vo_freq/1 -> Gain1/1
  vo_ampl/1 -> v_beta/1, v_alpha/1
  Subsystem1/1(ioa) -> Rate Transition11/1
  Subsystem1/2(iob) -> Rate Transition12/1
  Subsystem1/3(ioc1) -> Rate Transition13/1
  Subsystem1/4(vi) -> Rate Transition14/1
  PROC_INT_BL1 - ninterrupt/1 -> Subsystem1/Trigger
  Rate Transition11/1 -> Mux/1
  Rate Transition12/1 -> Mux/2
  Rate Transition13/1 -> Mux/3
  Rate Transition14/1 -> abc to Alpha-Beta-Zero/1

== system SVM_test2/Function-Call Subsystem ==
  vo_alpha : Inport
  vo_beta : Inport  Port=2
  phi : Inport  Port=3
  vi_angle : Inport  Port=4
  vi_peak : Inport  Port=5
  function : TriggerPort  TriggerType=function-call  VariantControl=Variant
  Add : Sum  OutDataTypeStr=Inherit: Inherit via back propagation
  Amplitude_calculator : Subsystem
  Divide1 : Product  Inputs=*/  OutDataTypeStr=Inherit: Inherit via back propagation
  MATLAB Function : MATLAB Function  TreatAsAtomicUnit=on
  MATLAB Function1 : MATLAB Function  TreatAsAtomicUnit=on
  MATLAB Function2 : MATLAB Function  TreatAsAtomicUnit=on
  d1 : Outport
  d2 : Outport  Port=2
  d3 : Outport  Port=3
  d4 : Outport  Port=4
  Kv : Outport  Port=5
  Ki : Outport  Port=6
  wires:
  MATLAB Function/2(Kv) -> Kv/1  "Kv"
  MATLAB Function1/2(Ki) -> Ki/1  "Ki"
  MATLAB Function2/3(d3) -> d3/1
  MATLAB Function2/2(d2) -> d2/1
  MATLAB Function2/4(d4) -> d4/1
  vi_peak/1 -> Divide1/2
  Divide1/1 -> MATLAB Function2/4(q)
  MATLAB Function2/1(d1) -> d1/1
  Amplitude_calculator/1(Out1) -> Divide1/1
  phi/1 -> MATLAB Function2/3(phi), Add/2
  vo_alpha/1 -> Amplitude_calculator/1(vo_alpha), MATLAB Function/1(vo_alpha)
  vi_angle/1 -> Add/1
  MATLAB Function/1(alpha_o) -> MATLAB Function2/1(alpha_o)  "alpha_o"
  Add/1 -> MATLAB Function1/1(beta)
  MATLAB Function1/1(beta_o) -> MATLAB Function2/2(beta_i)  "beta_i"
  vo_beta/1 -> MATLAB Function/2(vo_beta), Amplitude_calculator/2(vo_beta)

== system SVM_test2/RTI Data ==
  RTI Data Store : Subsystem  Tag="struct('public',struct('sub',struct('name',{{'SVM_test2'}},'data',{{struct('TH',struct('thTaskInfo',struct('taskType',{'TIMER','HWINT','TMRINT','SWINT','GLINT'},'tasksNumOf',{1,2,0,0,0},'srcIds',{{'TIMERA'},{'FPGACL1FPGA_INTP0Ch0','FPGACL1FPGA_INTP0Ch1'},{},{},{}},'taskNames',{{['Timer Task 1']},{['PROC_INT_BL1 - interrupt'],['PROC_INT_BL1 - ninterrupt']},{},{},{}})),'th_tc',struct('dataType',{'TASK','TASK','TASK'},'taskGroupId',{'','',''},'taskGroupList',{{},{},{}},'taskSchedulingPolicy',{'FCFS','FCFS','FCFS'},'taskType',{'TIMER','HWINT','HWINT'},'blkh',{-1,['SVM_test2/PROC_INT_BL1 - interrupt/Common Hardware' char(10) 'Interrupt Interface'],['SVM_test2/PROC_INT_BL1 - ninterrupt/Common Hardware' char(10) 'Interrupt Interface']},'srcId',{'TIMERA','FPGACL1FPGA_INTP0Ch0','FPGACL1FPGA_INTP0Ch1'},'srcSgnName',{['Timer A interrupt'],['FPGA Type CL1 FPGA_INT Port 0 Channel 0'],['FPGA Type CL1 FPGA_INT Port 0 Channel 1']},'srcCpuName',{'','',''},'taskName',{['Timer Task 1  [0.002] s'],['PROC_INT_BL1 - interrupt'],['PROC_INT_BL1 - ninterrupt']},'taskNameDisplayExt',{'','',''},'smplTime',{0.002,0,0},'smplTimeOffs',{0,0,0},'hasFixedPriority',{0,0,0},'priority',{3,1,2},'hasFixedOvc',{0,0,0},'ovcType',{1,1,1},'ovcMax',{1,1,1}),'tc_th',struct('dataType',{'TASK','TASK','TASK'},'taskGroupId',{'','',''},'taskGroupList',{{},{},{}},'taskSchedulingPolicy',{'FCFS','FCFS','FCFS'},'taskType',{'TIMER','HWINT','HWINT'},'blkh',{-1,['SVM_test2/PROC_INT_BL1 - interrupt/Common Hardware' char(10) 'Interrupt Interface'],['SVM_test2/PROC_INT_BL1 - ninterrupt/Common Hardware' char(10) 'Interrupt Interface']},'srcId',{'TIMERA','FPGACL1FPGA_INTP0Ch0','FPGACL1FPGA_INTP0Ch1'},'srcSgnName',{['Timer A interrupt'],['FPGA Type CL1 FPGA_INT Port 0 Channel 0'],['FPGA Type CL1 FPGA_INT Port 0 Channel 1']},'srcCpuName',{'','',''},'taskName',{['Timer Task 1  [0.002] s'],['PROC_INT_BL1 - interrupt'],['PROC_INT_BL1 - ninterrupt']},'taskNameDisplayExt',{'','',''},'smplTime',{0.002,0,0},'smplTimeOffs',{0,0,0},'hasFixedPriority',{0,0,0},'priority',{3,1,2},'hasFixedOvc',{0,0,0},'ovcType',{1,1,1},'ovcMax',{1,1,1}))}})),'private',struct('version',struct('dsVer',uint32(2)),'access',struct('modified',['04-Dec-2024 20:53:27'],'type','Model','isPerm',1)))"  mask(RTI_DATA_STORE){}
      mask help:
      | RTI Data Store Block. This block is used by RTI to store internal model dependent data. Deleting this block will result in data loss.
      |
      | NEVER DELETE, COPY, OR MODIFY THIS BLOCK!
      mask Help:
      | RTI Data Store Block. This block is used by RTI to store internal model dependent data. Deleting this block will result in data loss.
      | 
      | NEVER DELETE, COPY, OR MODIFY THIS BLOCK!
      mask Display: text(0.5, 0.5, ' ', 'HorizontalAlignment', 'center');
